simulink model "HelloLamp"  (R2022a)
settings: Solver=VariableStepAuto  StartTime=0.0  StopTime=inf  RelTol=1e-3
settings Model: Creator=uie82234  LastModifiedBy=uie82234

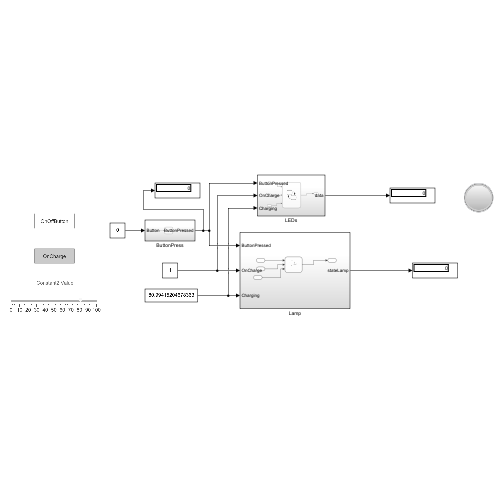
[thumbnail: Simulink's stored preview of the top-level diagram]
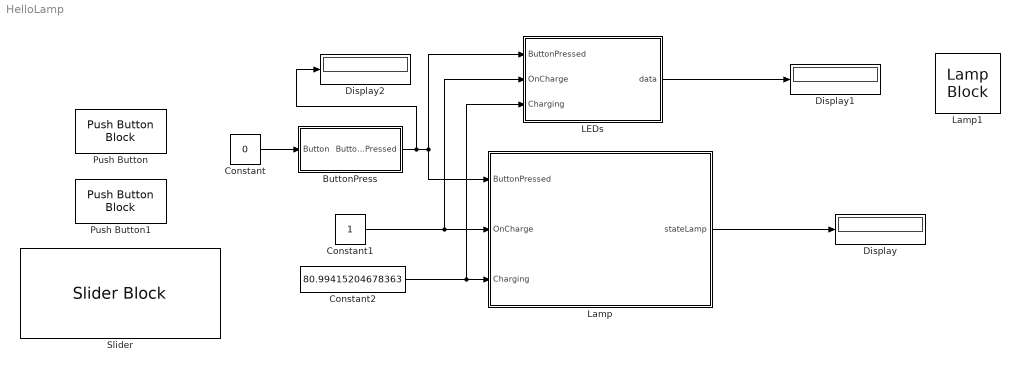
== system HelloLamp ==
  ButtonPress : Subsystem
  Constant : Constant  Value=0
  Constant1 : Constant
  Constant2 : Constant  Value=80.99415204678363
  Display : Display
  Display1 : Display
  Display2 : Display
  LEDs : Subsystem
  Lamp : Subsystem
  Lamp1 : LampBlock  LabelPosition=Hide
  Push Button : PushButtonBlock  ButtonText=OnOffButton  OffValue=0.000000
  Push Button1 : PushButtonBlock  ButtonText=OnCharge  ButtonType=Latch  OffValue=0.000000
  Slider : SliderBlock
  wires:
  Constant/1 -> ButtonPress/1(Button)
  Constant1/1 -> LEDs/2(OnCharge), Lamp/2(OnCharge)
  Constant2/1 -> LEDs/3(Charging), Lamp/3(Charging)
  Lamp/1(stateLamp) -> Display/1
  LEDs/1(data) -> Display1/1
  ButtonPress/1(ButtonPressed) -> Display2/1, Lamp/1(ButtonPressed), LEDs/1(ButtonPressed)

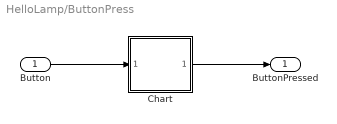
== system HelloLamp/ButtonPress ==
  Button : Inport
  Chart : Stateflow chart  TreatAsAtomicUnit=on
  ButtonPressed : Outport
  wires:
  Button/1 -> Chart/1(Button)
  Chart/1(ButtonPressed) -> ButtonPressed/1

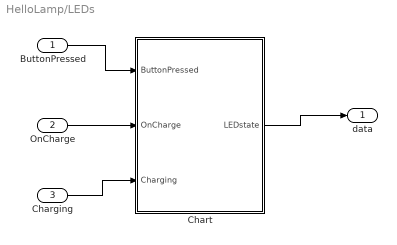
== system HelloLamp/LEDs ==
  ButtonPressed : Inport
  OnCharge : Inport  Port=2
  Charging : Inport  Port=3
  Chart : Stateflow chart  TreatAsAtomicUnit=on
  data : Outport
  wires:
  ButtonPressed/1 -> Chart/1(ButtonPressed)
  OnCharge/1 -> Chart/2(OnCharge)
  Charging/1 -> Chart/3(Charging)
  Chart/1(LEDstate) -> data/1

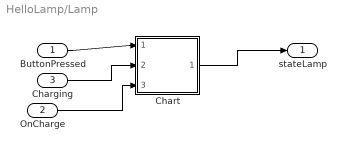
== system HelloLamp/Lamp ==
  ButtonPressed : Inport
  OnCharge : Inport  Port=2
  Charging : Inport  Port=3
  Chart : Stateflow chart  TreatAsAtomicUnit=on
  stateLamp : Outport
  wires:
  ButtonPressed/1 -> Chart/1(ButtonPressed)
  Charging/1 -> Chart/2(Charging)
  Chart/1(stateLamp) -> stateLamp/1
  OnCharge/1 -> Chart/3(OnCharge)

== stateflow chart HelloLamp/Lamp/Chart ==
  state On
    (history)
    state Low
      entry:
      stateLamp=1;
    state High
      entry:
      stateLamp=2;
    (default) -> Low
    High -> Low : [ButtonPressed == 1 || Charging < 60]
    Low -> High : [ButtonPressed == 1]
  state Off
    entry:
    stateLamp=0;
  (default) -> Off
  Off -> On : [ButtonPressed == 1]
  On -> Off : [ButtonPressed == 2 || Charging  < 20 || OnCharge == 1]
  data: ButtonPressed input; Charging input; stateLamp output; OnCharge input

== stateflow chart HelloLamp/LEDs/Chart ==
  state Red
    entry:
    LEDstate = 1;
  state Off
    entry:
    LEDstate = 0;
  state Yellow
    entry:
    LEDstate = 2;
  state Green
    entry:
    LEDstate = 3;
  (junction 10) -> Red [order 2] : [Charging <= 20]
  Red -> (junction 30)
  (default) -> Off
  Off -> (junction 10) : [ButtonPressed == 1 || (OnCharge == 1 && after(1,sec))]
  (junction 10) -> Yellow [order 1] : [Charging > 20 && Charging <=60]
  Yellow -> (junction 30)
  (junction 30) -> Off : after(1,sec)
  Green -> (junction 30)
  (junction 10) -> Green [order 3] : [Charging >60]
  (default) -> (junction 48) [commented out] : % Blink If Charging
  (junction 48) -> (junction 49) [commented out] : [OnCharge==1]
  (junction 48) -> (junction 50) [commented out]
  (junction 49) -> (junction 51) [commented out] : after(1,sec)
  (junction 51) -> (junction 50) [commented out]
  (junction 50) -> (junction 52) [commented out]
  data: ButtonPressed input; OnCharge input; Charging input; LEDstate output

== stateflow chart HelloLamp/ButtonPress/Chart ==
  state Off
    entry:
    ButtonPressed =0;
  state Press
  state ShortPress
    entry:
    ButtonPressed=1;
  state LongPress
    entry:
    ButtonPressed = 2;
  ShortPress -> Off
  (default) -> Off
  Off -> Press : [hasChangedTo(Button,1)]
  Press -> ShortPress [order 1] : [hasChangedTo(Button, 0)]
  LongPress -> Off
  Press -> LongPress [order 2] : [after(2,sec) && Button ==1]
  data: Button input; ButtonPressed output
